simulink model "vertical_smm_3d_with_xz_lqr"  (R2015a)
settings: Solver=FixedStepDiscrete  SolverMode=SingleTasking  StartTime=0.0  StopTime=inf  FixedStep=sample_time  RelTol=1e-3
values from neighbouring files (symbols this model uses):
  forward_dx_of_dxstar = [-1.33773437568 -1.28773437515 -1.23773437461 -1.18773437408 -1.13773437355 -1.08773437301 -1.03773437248 -0.987734371946 -0.937734371413 -0.887734370879 -0.837734370532 -0.787734370254 ... (27552 elements, 41x21x32)]    [ref_trajs.mat]
  forward_x_of_dxstar = [0.243075305346 0.235858801492 0.228642297639 0.221425793786 0.214209289933 0.206992786079 0.199776282226 0.192559778373 0.18534327452 0.178126770666 0.17091026684 0.163693763058 ... (27552 elements, 41x21x32)]    [ref_trajs.mat]
  target_dx_range = [-1 -0.95 -0.9 -0.85 -0.8 -0.75 -0.7 -0.65 -0.6 -0.55 -0.5 -0.45 ... (41 elements, 1x41)]    [ref_trajs.mat]
undefined symbols (not defined in the file or in its folder): A1_notch_f1, A2_notch_f1, A_kalman_fourbar_gear, A_kalman_swing_load, A_kalman_transverse, A_kalman_vertical, A_lpf_accelerometer, A_lpf_dtau, A_lpf_fourbar_angles, A_lpf_imu, A_lpf_lateral_angle, B1_lpf_accelerometer, B1_lpf_dtau, B1_lpf_fourbar_angles, B1_lpf_imu, B1_lpf_lateral_angle, B1_notch_f1, B2_lpf_accelerometer, B2_lpf_dtau, B2_lpf_fourbar_angles, B2_lpf_imu, B2_lpf_lateral_angle, B2_notch_f1, B_dx_versus_x0, B_kalman_fourbar_gear, B_kalman_swing_load, B_kalman_transverse, B_kalman_vertical, backwards_K_sag_of_t, backwards_P_sag_of_t, C_kalman_fourbar_gear, C_kalman_swing_load, C_kalman_transverse, C_kalman_vertical, com_leg_motor, com_torso, contact_threshold, control_start_time, d_ankle_to_foot, d_vertical_com, desired_com_forward_velocity, desired_com_lateral_velocity, desired_initial_leg_roll_left, desired_initial_leg_roll_right, desired_stance_beta2, desired_standing_torso_pitch, desired_standing_torso_roll, desired_standing_z, desired_torso_pitch, desired_torso_roll, Discrete, enable_bouncing, fcut_contact, fdesignblkfcn, g, gcbh, HIP_MTR_MAX_CONT_TORQUE, HIP_MTR_MAX_TORQUE, i_leg_motor, i_robot ... (+91)
libraries: simulink x33, ctrlSharedLib x11, dsparch4 x10, dspfdesign x2
(part 5 of 7)

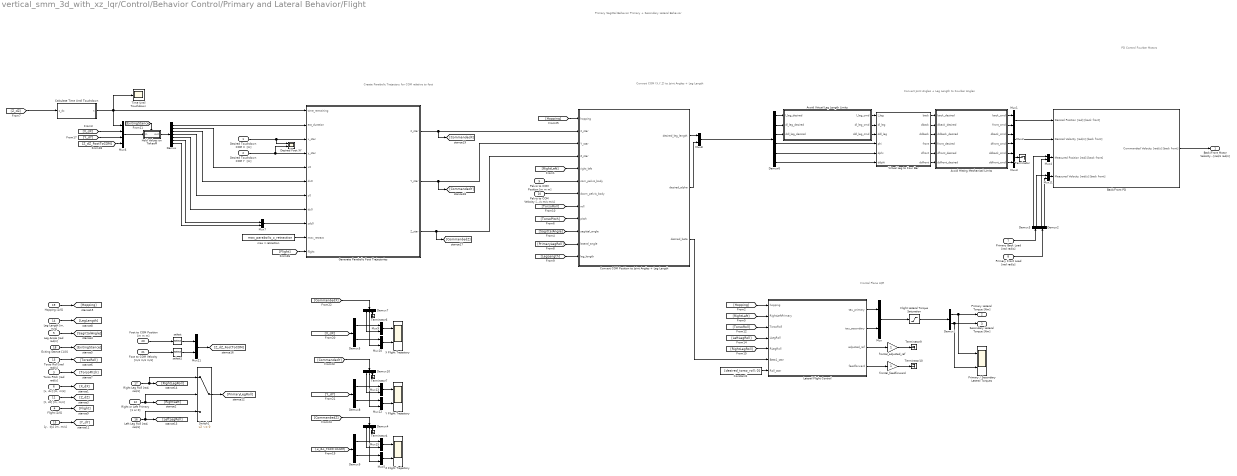
== system vertical_smm_3d_with_xz_lqr/Control/Behavior Control/Primary and Lateral Behavior/Flight ==
  note: Frontal Plane LQR
  note: PD Control Fourbar Motors
  note: Convert Joint Angles + Leg Length
      | to Fourbar Angles
  note: Convert COM (X,Y,Z) to
      | Joint Angles + Leg Length
  note: Create Parabolic
      | Trajectory for COM relative to foot
  note: Primary Sagittal Behavior
      | Primary + Secondary Lateral Behavior
  Desired Touchdown COM X  [m] : Inport
  Desired Touchdown COM Y  [m] : Inport  Port=2
  Torso Pitch [rad rad/s] : Inport  Port=3
  Flight [1/0] : Inport  Port=4
  Leg Angle [rad rad/s] : Inport  Port=5
  "[x, dx] [m, m/s]" : Inport  Port=6
  Primary Back Load [rad rad/s] : Inport  Port=7
  Primary Front Load [rad rad/s] : Inport  Port=8
  Pelvis to COM Position [m m m] : Inport  Port=9
  Pelvis to COM Velocity [m/s m/s m/s] : Inport  Port=10
  "[z, dz] [m, m/s]" : Inport  Port=11
  Right or Left Primary [1 or 0] : Inport  Port=12
  Torso Roll [rad rad/s] : Inport  Port=13
  "Leg Length [m, m/s]" : Inport  Port=14
  "[y,  dy] [m, m/s]" : Inport  Port=15
  "Left Leg Roll [rad, rad/s]" : Inport  Port=16
  "Right Leg Roll [rad, rad/s]" : Inport  Port=17
  Exiting Stance [1/0] : Inport  Port=18
  Hopping [1/0] : Inport  Port=19
  Foot to COM Position [m m m] : Inport  Port=20
  Foot to COM Velocity [m/s m/s m/s] : Inport  Port=21
  Avoid Hitting Mechanical Limits : MATLAB Function  TreatAsAtomicUnit=on
  Avoid Virtual Leg Length Limits : MATLAB Function  TreatAsAtomicUnit=on
  Back/Front PD : Subsystem
  Calculate Time Until Touchdown : MATLAB Function  TreatAsAtomicUnit=on
  Constant1 : Constant  Value=[desired_torso_roll; 0]
  "Convert COM Position to Joint Angles + Leg Length " : MATLAB Function  TreatAsAtomicUnit=on
  Demux : Demux  Outputs=7
  Demux{1..3,5,8..9} (6 alike) : Demux  Outputs=2
  Demux10 : Demux  Outputs=3
  Demux4 : Demux  Outputs=3
  Demux6 : Demux  Outputs=6
  Demux7 : Demux  Outputs=3
  Desired Foot XY : Scope  NumInputPorts=2
      settings: YMin=-1~-0.8  YMax=1~1.4  SaveName=ScopeData38  SampleInput=on
  Flight Lateral Torque Saturation : Saturate  UpperLimit=HIP_MTR_MAX_CONT_TORQUE  LowerLimit=-HIP_MTR_MAX_CONT_TORQUE
      settings: AttributesFormatString=Top: %<UpperLimit>\nBottom: %<LowerLimit>
  Generate Parabolic Foot Trajectories : MATLAB Function  TreatAsAtomicUnit=on
  Hold Values on Takeoff : Subsystem
  Lateral Flight Control : MATLAB Function  TreatAsAtomicUnit=on
  Mux{,1..5,7..13,15,21} (15 alike) : Mux  Inputs=2
  Mux6 : Mux
  Primary / Secondary Lateral Torques : Scope  NumInputPorts=2
      settings: YMin=-1~-0.8  YMax=1~1.4  SaveName=ScopeData32  SampleInput=on
  Switch1 : Switch  Criteria=u2 ~= 0
  Terminator{,4,6..7,9..10} (6 alike) : Terminator
  Time Until Touchdown : Scope
      settings: YMin=-1  YMax=1  SaveName=ScopeData37  SampleInput=on
  Virtual Leg to Four Bar : MATLAB Function  TreatAsAtomicUnit=on
  X Flight Trajectory : Scope  NumInputPorts=2
      settings: YMin=-1~-0.8  YMax=1~1.4  SaveName=ScopeData3  SampleInput=on
  Y Flight Trajectory : Scope  NumInputPorts=2
      settings: YMin=-1~-0.8  YMax=1~1.4  SaveName=ScopeData4  SampleInput=on
  Z Flight Trajectory : Scope  NumInputPorts=2
      settings: YMin=-1~-0.8  YMax=1~1.4  SaveName=ScopeData7  SampleInput=on
  frontal_adjusted_ref : Gain
  frontal_feedforward : Gain
  max z retraction : Constant  Value=max_parabolic_z_retraction
  select : Selector  InputPortWidth=3  Indices=[3]
  select1 : Selector  InputPortWidth=3  Indices=[3]
  Back/Front Motor Velocity [rad/s rad/s] : Outport
  Primary Lateral Torque [Nm] : Outport  Port=2
  Secondary Lateral Torque [Nm] : Outport  Port=3
  wires:
  Mux3/1 -> Terminator/1
  Generate Parabolic Foot Trajectories/3(Z_star) -> [CommandedZ], "Convert COM Position to Joint Angles + Leg Length "/4(Z_star)
  [CommandedZ] -> Demux4/1
  [CommandedY] -> Demux10/1
  [CommandedX] -> Demux7/1
  Demux10/3 -> Terminator7/1
  [Y_dY] -> Demux8/1
  Demux10/2 -> Mux12/2
  Demux10/1 -> Mux13/2
  Demux8/2 -> Mux12/1
  Demux8/1 -> Mux13/1
  Mux12/1 -> Y Flight Trajectory/2
  Mux13/1 -> Y Flight Trajectory/1
  Demux7/3 -> Terminator6/1
  [X_dX] -> Demux5/1
  Demux7/2 -> Mux10/2
  Demux7/1 -> Mux9/2
  Demux5/2 -> Mux10/1
  Demux5/1 -> Mux9/1
  Mux10/1 -> X Flight Trajectory/2
  Mux9/1 -> X Flight Trajectory/1
  Demux4/3 -> Terminator4/1
  Demux4/2 -> Mux5/2
  Demux4/1 -> Mux15/2
  Demux9/2 -> Mux5/1
  Demux9/1 -> Mux15/1
  [Z_dZ_FootToCOM] -> Demux9/1
  [Z_dZ_FootToCOM] -> Mux6/4
  Mux5/1 -> Z Flight Trajectory/2
  Mux15/1 -> Z Flight Trajectory/1
  Mux21/1 -> [Z_dZ_FootToCOM]
  select1/1 -> Mux21/2
  select/1 -> Mux21/1
  Foot to COM Velocity [m/s m/s m/s]/1 -> select1/1
  Foot to COM Position [m m m]/1 -> select/1
  Demux/7 -> Mux7/2
  Demux/6 -> Mux7/1
  Demux/5 -> Generate Parabolic Foot Trajectories/8(dy0)
  Demux/4 -> Generate Parabolic Foot Trajectories/7(y0)
  Demux/3 -> Generate Parabolic Foot Trajectories/6(dx0)
  Demux/2 -> Generate Parabolic Foot Trajectories/5(x0)
  [Flight] -> Generate Parabolic Foot Trajectories/11(flight)
  Hopping [1/0]/1 -> [Hopping]
  [Hopping] -> Lateral Flight Control/1(hopping)
  Mux/1 -> Flight Lateral Torque Saturation/1
  [Hopping] -> "Convert COM Position to Joint Angles + Leg Length "/1(hopping)
  frontal_adjusted_ref/1 -> Terminator9/1
  frontal_feedforward/1 -> Terminator10/1
  Flight Lateral Torque Saturation/1 -> Demux1/1
  "Convert COM Position to Joint Angles + Leg Length "/3(desired_beta) -> Lateral Flight Control/6(Beta1_star)
  Demux1/2 -> Secondary Lateral Torque [Nm]/1, Primary / Secondary Lateral Torques/2
  Demux1/1 -> Primary Lateral Torque [Nm]/1, Primary / Secondary Lateral Torques/1
  Exiting Stance [1/0]/1 -> [ExitingStance]
  Switch1/1 -> [PrimaryLegRoll]
  Right or Left Primary [1 or 0]/1 -> [RightLeft], Switch1/2
  "Right Leg Roll [rad, rad/s]"/1 -> [RightLegRoll], Switch1/1
  [RightLegRoll] -> Lateral Flight Control/5(RLegRoll)
  [LeftLegRoll] -> Lateral Flight Control/4(LLegRoll)
  "Left Leg Roll [rad, rad/s]"/1 -> [LeftLegRoll], Switch1/3
  Lateral Flight Control/1(tau_primary) -> Mux/1
  Lateral Flight Control/2(tau_secondary) -> Mux/2
  Lateral Flight Control/4(feedforward) -> frontal_feedforward/1
  Lateral Flight Control/3(adjusted_ref) -> frontal_adjusted_ref/1
  Constant1/1 -> Lateral Flight Control/7(Roll_star)
  [TorsoRoll] -> Lateral Flight Control/3(TorsoRoll)
  [RightLeft] -> Lateral Flight Control/2(RightLeftPrimary)
  Desired Touchdown COM Y  [m]/1 -> Generate Parabolic Foot Trajectories/4(y_star), Desired Foot XY/2
  Demux6/3 -> Avoid Virtual Leg Length Limits/3(ddl_leg_desired)
  Demux6/2 -> Avoid Virtual Leg Length Limits/2(dl_leg_desired)
  Demux6/1 -> Avoid Virtual Leg Length Limits/1(l_leg_desired)
  Avoid Virtual Leg Length Limits/3(ddl_leg_cmd) -> Virtual Leg to Four Bar/3(ddl_leg)
  Avoid Virtual Leg Length Limits/2(dl_leg_cmd) -> Virtual Leg to Four Bar/2(dl_leg)
  Avoid Virtual Leg Length Limits/1(l_leg_cmd) -> Virtual Leg to Four Bar/1(l_leg)
  Calculate Time Until Touchdown/1(t) -> Generate Parabolic Foot Trajectories/1(time_remaining), Time Until Touchdown/1, Mux6/1
  [Z_dZ] -> Calculate Time Until Touchdown/1(z_dz)
  [Y_dY] -> Mux6/3
  "[y,  dy] [m, m/s]"/1 -> [Y_dY]
  Desired Touchdown COM X  [m]/1 -> Generate Parabolic Foot Trajectories/3(x_star), Desired Foot XY/1
  "[z, dz] [m, m/s]"/1 -> [Z_dZ]
  "Leg Length [m, m/s]"/1 -> [LegLength]
  Torso Roll [rad rad/s]/1 -> [TorsoRoll]
  "[x, dx] [m, m/s]"/1 -> [X_dX]
  [ExitingStance] -> Hold Values on Takeoff/Trigger
  Flight [1/0]/1 -> [Flight]
  Pelvis to COM Velocity [m/s m/s m/s]/1 -> "Convert COM Position to Joint Angles + Leg Length "/7(dcom_pelvis_body)
  Pelvis to COM Position [m m m]/1 -> "Convert COM Position to Joint Angles + Leg Length "/6(com_pelvis_body)
  [TorsoRoll] -> "Convert COM Position to Joint Angles + Leg Length "/8(roll)
  [LegLength] -> "Convert COM Position to Joint Angles + Leg Length "/12(leg_length)
  [PrimaryLegRoll] -> "Convert COM Position to Joint Angles + Leg Length "/11(lateral_angle)
  [TorsoPitch] -> "Convert COM Position to Joint Angles + Leg Length "/9(pitch)
  Torso Pitch [rad rad/s]/1 -> [TorsoPitch]
  [SagittalAngle] -> "Convert COM Position to Joint Angles + Leg Length "/10(sagittal_angle)
  Leg Angle [rad rad/s]/1 -> [SagittalAngle]
  Mux8/1 -> Demux6/1
  Demux6/4 -> Virtual Leg to Four Bar/4(phi)
  Demux6/5 -> Virtual Leg to Four Bar/5(dphi)
  Demux6/6 -> Virtual Leg to Four Bar/6(ddphi)
  "Convert COM Position to Joint Angles + Leg Length "/1(desired_leg_length) -> Mux8/1
  "Convert COM Position to Joint Angles + Leg Length "/2(desired_alpha) -> Mux8/2
  [RightLeft] -> "Convert COM Position to Joint Angles + Leg Length "/5(right_left)
  Generate Parabolic Foot Trajectories/2(Y_star) -> [CommandedY], "Convert COM Position to Joint Angles + Leg Length "/3(Y_star)
  Generate Parabolic Foot Trajectories/1(X_star) -> "Convert COM Position to Joint Angles + Leg Length "/2(X_star), [CommandedX]
  [X_dX] -> Mux6/2
  Hold Values on Takeoff/1(out) -> Demux/1
  Mux6/1 -> Hold Values on Takeoff/1(in)
  max z retraction/1 -> Generate Parabolic Foot Trajectories/10(max_retract)
  Mux7/1 -> Generate Parabolic Foot Trajectories/9(zdz0)
  Demux/1 -> Generate Parabolic Foot Trajectories/2(est_duration)
  Primary Front Load [rad rad/s]/1 -> Demux2/1
  Primary Back Load [rad rad/s]/1 -> Demux3/1
  Back/Front PD/1(Commanded Velocity [rad/s] [back front]) -> Back/Front Motor Velocity [rad/s rad/s]/1
  Mux2/1 -> Back/Front PD/2(Desired Velocity [rad/s] [back front])
  Avoid Hitting Mechanical Limits/6(ddfront_cmd) -> Mux3/2
  Avoid Hitting Mechanical Limits/5(ddback_cmd) -> Mux3/1
  Avoid Hitting Mechanical Limits/4(dfront_cmd) -> Mux2/2
  Avoid Hitting Mechanical Limits/3(dback_cmd) -> Mux2/1
  Demux2/1 -> Mux4/2
  Avoid Hitting Mechanical Limits/1(back_cmd) -> Mux1/1
  Avoid Hitting Mechanical Limits/2(front_cmd) -> Mux1/2
  Demux3/1 -> Mux4/1
  Demux3/2 -> Mux11/1
  Mux1/1 -> Back/Front PD/1(Desired Position [rad] [back front])
  Mux4/1 -> Back/Front PD/3(Measured Position [rad] [back front])
  Demux2/2 -> Mux11/2
  Mux11/1 -> Back/Front PD/4(Measured Velocity [rad/s] [back front])
  Virtual Leg to Four Bar/6(ddfront) -> Avoid Hitting Mechanical Limits/6(ddfront_desired)
  Virtual Leg to Four Bar/5(dfront) -> Avoid Hitting Mechanical Limits/5(dfront_desired)
  Virtual Leg to Four Bar/4(front) -> Avoid Hitting Mechanical Limits/4(front_desired)
  Virtual Leg to Four Bar/3(ddback) -> Avoid Hitting Mechanical Limits/3(ddback_desired)
  Virtual Leg to Four Bar/2(dback) -> Avoid Hitting Mechanical Limits/2(dback_desired)
  Virtual Leg to Four Bar/1(back) -> Avoid Hitting Mechanical Limits/1(back_desired)

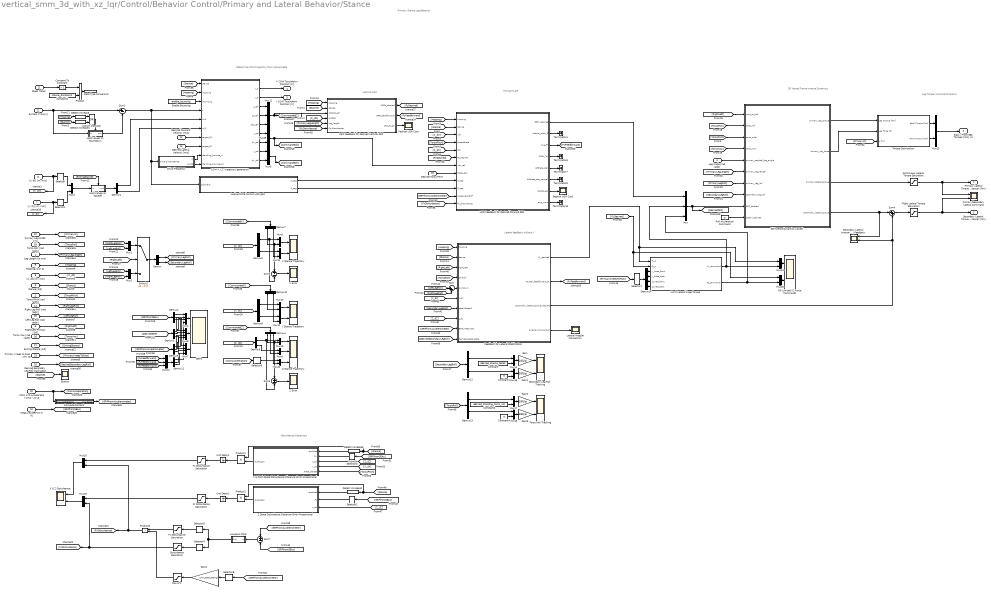
== system vertical_smm_3d_with_xz_lqr/Control/Behavior Control/Primary and Lateral Behavior/Stance ==
  note: Leg Torque / Force
      | Distribution
  note: Disturbance Observers
  note: Primary Stance Leg Behavior
  note: Determine COM trajectory
      | from lookup table
  note: Vertical LQR
  note: Forward LQR
  note: 3D Yawed Frame Inverse Dynamics
  note: Lateral feedback without Y
  Leg Length [m m/s] : Inport
  Torso Pitch [rad rad/s] : Inport  Port=2
  Stance [1/0] : Inport  Port=3
  Leg Angle [rad rad/s] : Inport  Port=4
  Right/Left Primary [1/0] : Inport  Port=5
  "[x, dx] [m, m/s]" : Inport  Port=6
  "[y, dy] [m, m/s]" : Inport  Port=7
  "[z, dz] [m, m/s]" : Inport  Port=8
  Hopping [1 or 0] : Inport  Port=9
  Measured GRF [N N N] : Inport  Port=10
  Steps Taken : Inport  Port=11
  Desired Forward Velocity [m/s] : Inport  Port=12
  Desired Lateral Velocity [m/s] : Inport  Port=13
  Right Leg Roll [rad rad/s] : Inport  Port=14
  Left Leg Roll [rad rad/s] : Inport  Port=15
  Torso Yaw [rad rad/s] : Inport  Port=16
  Exiting Stance [1/0] : Inport  Port=17
  Desired Torso Pitch : Inport  Port=18
  Torso Roll [rad rad/s] : Inport  Port=19
  COM XYZ Acceleration [m/s^2] x3 : Inport  Port=20
  System Time [s] : Inport  Port=21
  Primary Leg Width [m] : Inport  Port=22
  Primary Knees to Foot [m] x6 : Inport  Port=23
  Desired Secondary Leg Roll [rad rad/s] : Inport  Port=24
  3D Inverse Dynamics yawed : MATLAB Function  TreatAsAtomicUnit=on
  COM X,Y,Z  trajectory generation : MATLAB Function  TreatAsAtomicUnit=on
  Chirp Frequency : Subsystem
  Compare To Constant : simulink/Logic and Bit Operations/Compare To Constant  relop=<  const=1  OutDataTypeStr=uint8
  Compute Forces1 : Subsystem
  Constant : Constant  Value=desired_stance_beta2
  Constant1 : Constant  Value=0
  Constant2 : Constant  Value=stance_duration/2
  Constant3 : Constant  Value=desired_standing_torso_roll
  Constant4 : Constant  Value=0
  Continuous Lateral Torque Saturation : Saturate  UpperLimit=max_primary_lateral_stance_torque  LowerLimit=-max_primary_lateral_stance_torque
      settings: AttributesFormatString=Top: %<UpperLimit>\nBottom: %<LowerLimit>
  Data Type Conversion : DataTypeConversion  OutDataTypeStr=double
  Demux{,1,5,7..10,12..13} (9 alike) : Demux  Outputs=2
  Demux{2..4,6,11} (5 alike) : Demux  Outputs=3
  Demux14 : Demux
  Detect Increase{,1..3} (4 alike) : simulink/Logic and Bit Operations/Detect Increase  vinit=0.0  InputProcessing=Inherited  OutDataTypeStr=boolean
  "Disturbance Saturation " : Saturate  UpperLimit=100  LowerLimit=-100
      settings: AttributesFormatString=Top: %<UpperLimit>\nBottom: %<LowerLimit>
  Enable Bouncing : Constant  Value=enable_bouncing  SampleTime=sample_time
  Feedback for Lateral Stabilization : MATLAB Function  TreatAsAtomicUnit=on
  Flight Lateral Torque Saturation : Saturate  UpperLimit=HIP_MTR_MAX_CONT_TORQUE  LowerLimit=-HIP_MTR_MAX_CONT_TORQUE
      settings: AttributesFormatString=Top: %<UpperLimit>\nBottom: %<LowerLimit>
  Fx Disturbance Saturation : Saturate  UpperLimit=100  LowerLimit=-100
      settings: AttributesFormatString=Top: %<UpperLimit>\nBottom: %<LowerLimit>
  "Fx Disturbance Saturation " : Saturate  UpperLimit=100  LowerLimit=-100
      settings: AttributesFormatString=Top: %<UpperLimit>\nBottom: %<LowerLimit>
  Fz Disturbance Saturation : Saturate  UpperLimit=100  LowerLimit=-100
      settings: AttributesFormatString=Top: %<UpperLimit>\nBottom: %<LowerLimit>
  GRFs : Scope  NumInputPorts=3
      settings: TimeRange=37.999  YMin=-1250~-2000~-1250  YMax=1500~3750~1750  SampleInput=on
  Gain{,1..3} (4 alike) : Gain  Gain=180/pi
  Gain4 : Gain  Gain=2/(m_total_real*g)
  Hold Values on Takeoff : Subsystem
  Hold Values on Touchdown : Subsystem
  LQR Feedback for Desired Forward GRF : MATLAB Function  TreatAsAtomicUnit=on
  LQR Feedback for Desired Vertical GRF : MATLAB Function  TreatAsAtomicUnit=on
  Lateral Angular Momentum : Scope
      settings: YMin=-3.5  YMax=4  SaveName=ScopeData20  SampleInput=on
  Limit Lateral Knee Torque : MATLAB Function  TreatAsAtomicUnit=on
  Logical Operator : Logic  Operator=OR  AllPortsSameDT=off  OutDataTypeStr=boolean
  Lookup finite horizon LQR gain : MATLAB Function  TreatAsAtomicUnit=on
  Lowpass Filter : Subsystem  DialogController=fdesignblkfcn  InitFcn=fdesignblkfcn(gcbh, {'InitFcn'});  mask(Lowpass Filter){}
      mask help: Design a lowpass filter
      settings: CopyFcn=fdesignblkfcn(gcbh, {'CopyFcn'});
      mask Help: helpview(mapfilelocation('dsp'), 'dsplowpassfilter');
      mask Display: disp('Lowpass')
  Max of 1 : Saturate  UpperLimit=1  LowerLimit=0
      settings: AttributesFormatString=Top: %<UpperLimit>\nBottom: %<LowerLimit>
  Mux : Mux  Inputs=3
  Mux{1..3,5,8..10,12..20,22..25,49} (21 alike) : Mux  Inputs=2
  Mux11 : Mux  Inputs=3
  Mux21 : Mux  Inputs=3
  Mux4 : Mux
  Mux6 : Mux
  Mux7 : Mux
  Primary/Secondary Lateral Command : Scope  NumInputPorts=2
      settings: YMin=40~-5  YMax=150~5  SaveName=ScopeData25  SampleInput=on
  Product{,1..3} (4 alike) : Product
  QP Limited YZ Force Commands : Scope  NumInputPorts=2
      settings: YMin=40~-5  YMax=150~5  SaveName=ScopeData26  SampleInput=on
  Roll Accleration Command : Constant  Value=0
  Sagittal LQR Cost : Scope
      settings: YMin=22.5  YMax=62.5  SaveName=ScopeData10  SampleInput=on
  Secondary Lateral Inverse Dynamics / Feedback : Scope  NumInputPorts=2
      settings: YMin=-3.5~-5  YMax=4~5  SaveName=ScopeData9  SampleInput=on
  Secondary Leg Roll Tracking : Scope  NumInputPorts=2
      settings: YMin=-3.5~-5  YMax=4~5  SaveName=ScopeData12  SampleInput=on
  Selector : Selector  InputPortWidth=2  Indices=[2]
  Selector1 : Selector  InputPortWidth=2  Indices=[2]
  Selector{2,4,6,8} (4 alike) : Selector  InputPortWidth=3  Indices=[3]
  Selector3 : Selector  InputPortWidth=3  Indices=[1]
  Selector5 : Selector  InputPortWidth=3  Indices=[1]
  Selector7 : Selector  InputPortWidth=6  Indices=[2 5 3 6]
  Stance : Scope
      settings: YMin=-0.05  YMax=0.11  SaveName=stance_time_history  SampleInput=on
  Sum : Sum  Inputs=|+-
  Sum2 : Sum  Inputs=|+-
  Sum4 : Sum  Inputs=|++
  Sum5 : Sum  Inputs=+-
  Sum6 : Sum  Inputs=+-
  Sum7 : Sum  Inputs=+-
  Switch1 : Switch  Criteria=u2 ~= 0
  Terminator{4,6..8,10} (5 alike) : Terminator
  Torque Distribution : Subsystem
  Torso Roll Tracking : Scope  NumInputPorts=2
      settings: YMin=-3.5~-5  YMax=4~5  SaveName=ScopeData15  SampleInput=on
  Unit Delay1 : UnitDelay  SampleTime=sample_time
  Unit Delay2 : UnitDelay  SampleTime=sample_time
  Vertical LQR Cost : Scope
      settings: YMin=11  YMax=16  SaveName=ScopeData18  SampleInput=on
  X & Pitch State Disturbance Observer Error-Proportional : MATLAB Function  TreatAsAtomicUnit=on
  X & Z Disturbance : Scope  NumInputPorts=2
      settings: YMin=-125~-800  YMax=175~700  SaveName=ScopeData16  SampleInput=on
  X Stance Trajectory : Scope  NumInputPorts=2
      settings: YMin=0~-0.02  YMax=0.005~0.03  SaveName=ScopeData8  SampleInput=on
  X error : Scope
      settings: YMin=-0.05  YMax=0.11  SaveName=ScopeData24  SampleInput=on
  Y Stance Trajectory : Scope  NumInputPorts=2
      settings: YMin=0.005~-0.5  YMax=0.1~0.3  SaveName=ScopeData5  SampleInput=on
  Z Error : Scope
      settings: YMin=-0.007  YMax=0.0005  SaveName=ScopeData23  SampleInput=on
  Z Stance Trajectory : Scope  NumInputPorts=3
      settings: YMin=0.85~-0.4~-3  YMax=0.98~0.6~11  SaveName=z_stance_trajectory  SampleInput=on
  Z State Disturbance Observer Error-Proportional : MATLAB Function  TreatAsAtomicUnit=on
  Primary Lateral Torque Command (stance) [Nm] : Outport
  Secondary Lateral Torque Command (stance) [Nm] : Outport  Port=2
  Back / Front SEA Torques [Nm] x2 : Outport  Port=3
  X COM Touchdown Position [m] : Outport  Port=4
  Y COM Touchdown Position [m] : Outport  Port=5
  wires:
  Limit Lateral Knee Torque/1(Fy_command) -> Mux/2, Mux24/2
  Mux25/1 -> QP Limited YZ Force Commands/2
  Mux24/1 -> QP Limited YZ Force Commands/1
  Selector7/1 -> Demux14/1
  Demux14/4 -> Limit Lateral Knee Torque/6(z_knee_back)
  Demux14/3 -> Limit Lateral Knee Torque/5(z_knee_front)
  Demux14/2 -> Limit Lateral Knee Torque/4(y_knee_back)
  Demux14/1 -> Limit Lateral Knee Torque/3(y_knee_front)
  [PrimaryKneesToFoot] -> Selector7/1
  Primary Knees to Foot [m] x6/1 -> [PrimaryKneesToFoot]
  Feedback for Lateral Stabilization/2(neutral_feedforward_Fy) -> [FyFeedforward]
  LQR Feedback for Desired Forward GRF/2(netural_pitch_ff) -> Terminator4/1
  LQR Feedback for Desired Forward GRF/3(true_ff) -> [FxFeedforward]
  Compute Forces1/1(XYZ Force) -> [GRFfromAccelerometer]
  [FyFeedforward] -> Mux21/2
  [Z_dZ] -> Feedback for Lateral Stabilization/8(z_dz)
  [FzDesired] -> Mux25/1, Limit Lateral Knee Torque/2(Fz_s)
  [FzDesired] -> LQR Feedback for Desired Forward GRF/6(Fz_desired)
  [FxFeedforward] -> Mux21/1
  Mux23/1 -> Back / Front SEA Torques [Nm] x2/1
  Torque Distribution/2(Front Torque [Nm]) -> Mux23/2
  Torque Distribution/1(Back Torque [Nm]) -> Mux23/1
  Primary Leg Width [m]/1 -> [PrimaryW]
  3D Inverse Dynamics yawed/2(primary_leg_force) -> Torque Distribution/2(Leg Force [N])
  [PrimaryW] -> Torque Distribution/3(w [m])
  3D Inverse Dynamics yawed/1(primary_leg_torque) -> Torque Distribution/1(Leg Torque [Nm])
  Selector6/1 -> Mux22/1
  [ComAcceleration] -> Selector6/1
  Mux22/1 -> Z Stance Trajectory/3
  Sum5/1 -> Z Error/1
  [CommandedZ] -> Demux4/1
  Demux4/3 -> Mux22/2
  Demux4/2 -> Mux8/2
  Demux4/1 -> Sum5/1, Mux15/2
  Demux9/2 -> Mux8/1
  Demux9/1 -> Sum5/2, Mux15/1
  [Z_dZ] -> Demux9/1
  Mux8/1 -> Z Stance Trajectory/2
  Mux15/1 -> Z Stance Trajectory/1
  [FzFeedforward] -> Mux21/3
  Mux21/1 -> Demux11/1
  LQR Feedback for Desired Vertical GRF/2(GRFz_feedforward) -> [FzFeedforward]
  [GRFfromAccelerometer] -> Demux6/1
  COM XYZ Acceleration [m/s^2] x3/1 -> [ComAcceleration], Compute Forces1/1(XYZ Acceleration)
  Selector4/1 -> "Disturbance Saturation "/1
  [GRFfromSEAs] -> Sum7/2
  Mux19/1 -> X & Z Disturbance/2
  [Stance] -> Detect Increase2/1, Product2/1
  Z State Disturbance Observer Error-Proportional/1(d_hat_tp1) -> Product2/2
  [Stance] -> Detect Increase3/1, Product1/1
  X & Pitch State Disturbance Observer Error-Proportional/1(d_hat_tp1) -> Product1/2
  Product2/1 -> Unit Delay2/1
  Product1/1 -> Unit Delay1/1
  [Z_dZ] -> Z State Disturbance Observer Error-Proportional/3(z_dz)
  [GRFfromSEAs] -> Selector2/1
  Detect Increase2/1 -> Z State Disturbance Observer Error-Proportional/1(enabled)
  Detect Increase3/1 -> X & Pitch State Disturbance Observer Error-Proportional/1(enabled)
  [GRFfromSEAs] -> Selector3/1
  [X_dX] -> X & Pitch State Disturbance Observer Error-Proportional/4(x_dx)
  [TorsoPitch] -> X & Pitch State Disturbance Observer Error-Proportional/5(theta_dtheta)
  [Z_dZ] -> X & Pitch State Disturbance Observer Error-Proportional/3(z_dz)
  "[z, dz] [m, m/s]"/1 -> [Z_dZ]
  Flight Lateral Torque Saturation/1 -> Secondary Lateral Torque Command (stance) [Nm]/1, Primary/Secondary Lateral Command/2
  Demux6/3 -> Mux7/3
  Demux6/2 -> Mux6/3
  Demux6/1 -> Mux4/3
  Feedback for Lateral Stabilization/4(angular_momentum) -> Lateral Angular Momentum/1
  LQR Feedback for Desired Forward GRF/4(GRFx_lqr) -> Terminator6/1
  [Stance] -> COM X,Y,Z  trajectory generation/1(stance)
  Lookup finite horizon LQR gain/2(P_sag) -> LQR Feedback for Desired Forward GRF/10(P_sag)
  [Z_dZ] -> LQR Feedback for Desired Vertical GRF/4(z_state)
  COM X,Y,Z  trajectory generation/3(z_ref) -> Mux11/1
  [Stance] -> LQR Feedback for Desired Forward GRF/2(stance)
  COM X,Y,Z  trajectory generation/6(x_ref) -> Mux49/1
  COM X,Y,Z  trajectory generation/7(dx_ref) -> Mux49/2
  COM X,Y,Z  trajectory generation/8(y_ref) -> Mux5/1
  COM X,Y,Z  trajectory generation/9(dy_ref) -> Mux5/2
  COM X,Y,Z  trajectory generation/1(x_0) -> X COM Touchdown Position [m]/1
  COM X,Y,Z  trajectory generation/4(dz_ref) -> Mux11/2
  COM X,Y,Z  trajectory generation/5(ddz_ref) -> Mux11/3
  Mux11/1 -> [CommandedZ], LQR Feedback for Desired Vertical GRF/3(zdzddz_ref)
  [X_dX] -> LQR Feedback for Desired Forward GRF/3(xdx)
  [TorsoPitch] -> LQR Feedback for Desired Forward GRF/4(thetadtheta)
  Mux49/1 -> [CommandedX], LQR Feedback for Desired Forward GRF/7(xdx_ref)
  Desired Torso Pitch/1 -> LQR Feedback for Desired Forward GRF/8(theta_star)
  Lookup finite horizon LQR gain/1(K_sag) -> LQR Feedback for Desired Forward GRF/9(K_sag)
  [Z_dZ] -> LQR Feedback for Desired Forward GRF/5(zdz)
  Desired Forward Velocity [m/s]/1 -> COM X,Y,Z  trajectory generation/7(target_DX)
  Sum2/1 -> COM X,Y,Z  trajectory generation/4(t), Lookup finite horizon LQR gain/1(t_forward), Chirp Frequency/1(Time Since Stance)
  LQR Feedback for Desired Vertical GRF/1(GRFz_desired) -> [FzDesired]
  Hold Values on Touchdown/1(out) -> Sum2/2
  Stance [1/0]/1 -> [Stance]
  [Stance] -> LQR Feedback for Desired Vertical GRF/2(stance)
  Logical Operator/1 -> Hold Values on Touchdown/Trigger
  "[x, dx] [m, m/s]"/1 -> [X_dX], Selector/1
  Demux1/2 -> COM X,Y,Z  trajectory generation/6(dy0)
  LQR Feedback for Desired Vertical GRF/3(cost_to_go) -> Vertical LQR Cost/1
  LQR Feedback for Desired Forward GRF/5(ddtheta_star) -> Terminator7/1
  LQR Feedback for Desired Forward GRF/6(ddtheta_star_neutral) -> Terminator8/1
  LQR Feedback for Desired Forward GRF/7(cost_to_go) -> Sagittal LQR Cost/1
  LQR Feedback for Desired Forward GRF/8(ang_mom) -> Terminator10/1
  Torso Pitch [rad rad/s]/1 -> [TorsoPitch]
  [RightLeft] -> 3D Inverse Dynamics yawed/1(right_or_left)
  Hopping [1 or 0]/1 -> [Hopping]
  [Hopping] -> COM X,Y,Z  trajectory generation/2(hopping)
  [Hopping] -> LQR Feedback for Desired Forward GRF/1(hopping)
  Measured GRF [N N N]/1 -> [GRFfromSEAs]
  [GRFfromAccelerometer] -> LQR Feedback for Desired Forward GRF/11(measured_GRF)
  Steps Taken/1 -> Compare To Constant/1
  Product/1 -> Data Type Conversion/1
  Constant2/1 -> Product/2
  Detect Increase/1 -> Logical Operator/1
  Detect Increase1/1 -> Logical Operator/2
  Compare To Constant/1 -> Product/1
  [Hopping] -> Detect Increase/1
  [Stance] -> Detect Increase1/1
  Demux1/1 -> COM X,Y,Z  trajectory generation/5(dx0)
  Selector/1 -> Mux3/1
  [Hopping] -> LQR Feedback for Desired Vertical GRF/1(hopping)
  [Stance] -> Feedback for Lateral Stabilization/2(stance)
  [TorsoRoll] -> Feedback for Lateral Stabilization/4(rolldroll)
  COM X,Y,Z  trajectory generation/2(y_0) -> Y COM Touchdown Position [m]/1
  Mux5/1 -> [CommandedY]
  [TorsoPitch] -> 3D Inverse Dynamics yawed/3(torso_pitch)
  [TorsoRoll] -> 3D Inverse Dynamics yawed/2(torso_roll)
  [TorsoYaw] -> 3D Inverse Dynamics yawed/4(torso_yaw)
  [PrimaryLegLength] -> 3D Inverse Dynamics yawed/6(primary_leg_length)
  Leg Angle [rad rad/s]/1 -> 3D Inverse Dynamics yawed/5(primary_sagittal_leg_angle)
  [SecondaryLegRoll] -> 3D Inverse Dynamics yawed/8(secondary_leg_roll)
  [PrimaryLegRoll] -> 3D Inverse Dynamics yawed/7(primary_leg_roll)
  Switch1/1 -> Demux/1
  Demux/2 -> [SecondaryLegRoll]
  Demux/1 -> [PrimaryLegRoll]
  Mux1/1 -> Switch1/1
  Mux2/1 -> Switch1/3
  Right Leg Roll [rad rad/s]/1 -> [RightLegRoll]
  [RightLegRoll] -> Mux1/1
  [LeftLegRoll] -> Mux1/2
  [LeftLegRoll] -> Mux2/1
  [RightLegRoll] -> Mux2/2
  [RightLeft] -> Switch1/2
  "[y, dy] [m, m/s]"/1 -> [Y_dY], Selector1/1
  Mux3/1 -> Hold Values on Takeoff/1(in)
  Hold Values on Takeoff/1(out) -> Demux1/1
  Selector1/1 -> Mux3/2
  Desired Lateral Velocity [m/s]/1 -> COM X,Y,Z  trajectory generation/8(target_DY)
  Torso Yaw [rad rad/s]/1 -> [TorsoYaw]
  Exiting Stance [1/0]/1 -> [ExitingStance]
  [ExitingStance] -> Hold Values on Takeoff/Trigger
  [Hopping] -> Feedback for Lateral Stabilization/1(hopping)
  [GRFfromAccelerometer] -> Feedback for Lateral Stabilization/9(GRF_measured)
  System Time [s]/1 -> Hold Values on Touchdown/1(in), Sum2/1
  Leg Length [m m/s]/1 -> [PrimaryLegLength]
  [PrimaryLegLength] -> LQR Feedback for Desired Vertical GRF/5(leg_length)
  Torso Roll [rad rad/s]/1 -> [TorsoRoll]
  [GRFfromSEAs] -> Demux2/1
  [DesiredGRF] -> Demux3/1
  Mux4/1 -> GRFs/1
  Demux2/1 -> Mux4/1
  Mux6/1 -> GRFs/2
  Mux7/1 -> GRFs/3
  Demux2/2 -> Mux6/1
  Demux2/3 -> Mux7/1
  Demux3/1 -> Mux4/2
  Demux3/2 -> Mux6/2
  Demux3/3 -> Mux7/2
  Mux9/1 -> X Stance Trajectory/1
  Mux10/1 -> X Stance Trajectory/2
  Demux5/2 -> Mux10/1
  Demux7/2 -> Mux10/2
  [X_dX] -> Demux5/1
  Mux13/1 -> Y Stance Trajectory/1
  Mux12/1 -> Y Stance Trajectory/2
  Demux8/1 -> Mux13/1
  Demux8/2 -> Mux12/1
  Demux10/1 -> Mux13/2
  Demux10/2 -> Mux12/2
  [Y_dY] -> Demux8/1
  [CommandedX] -> Demux7/1
  [CommandedY] -> Demux10/1
  Right/Left Primary [1/0]/1 -> [RightLeft]
  Left Leg Roll [rad rad/s]/1 -> [LeftLegRoll]
  LQR Feedback for Desired Forward GRF/1(GRFx_desired) -> Mux/1
  Mux/1 -> 3D Inverse Dynamics yawed/9(GRF_desired), [DesiredGRF]
  Demux11/1 -> Mux4/4
  Demux11/2 -> Mux6/4
  Demux11/3 -> Mux7/4
  Continuous Lateral Torque Saturation/1 -> Primary Lateral Torque Command (stance) [Nm]/1, Primary/Secondary Lateral Command/1
  Feedback for Lateral Stabilization/1(Fy_desired) -> Mux24/1, Limit Lateral Knee Torque/1(Fy_s)
  Roll Accleration Command/1 -> 3D Inverse Dynamics yawed/10(ddRoll_desired)
  [LeftLegRoll] -> Sum/1
  [RightLegRoll] -> Sum/2
  [Y_dY] -> Feedback for Lateral Stabilization/6(y_dy)
  [SecondaryLegRoll] -> Feedback for Lateral Stabilization/7(beta2dbeta2)
  Sum/1 -> Feedback for Lateral Stabilization/5(symdsym)
  3D Inverse Dynamics yawed/4(secondary_lateral_torque) -> Sum4/1, Secondary Lateral Inverse Dynamics / Feedback/1
  3D Inverse Dynamics yawed/3(primary_lateral_torque) -> Continuous Lateral Torque Saturation/1
  Sum4/1 -> Flight Lateral Torque Saturation/1
  Feedback for Lateral Stabilization/3(secondary_lateral_torque_desired) -> Secondary Lateral Inverse Dynamics / Feedback/2, Sum4/2
  [SecondaryLegRoll] -> Demux12/1
  Mux14/1 -> Gain/1
  Demux12/1 -> Mux14/1
  Constant/1 -> Mux14/2
  Gain/1 -> Secondary Leg Roll Tracking/1
  Gain1/1 -> Secondary Leg Roll Tracking/2
  Mux16/1 -> Gain1/1
  Demux12/2 -> Mux16/1
  Constant1/1 -> Mux16/2
  [TorsoRoll] -> Demux13/1
  Gain2/1 -> Torso Roll Tracking/1
  Gain3/1 -> Torso Roll Tracking/2
  Mux17/1 -> Gain2/1
  Demux13/1 -> Mux17/1
  Constant3/1 -> Mux17/2
  Demux13/2 -> Mux18/1
  Mux18/1 -> Gain3/1
  Constant4/1 -> Mux18/2
  [RightLeft] -> Feedback for Lateral Stabilization/3(right_left)
  Enable Bouncing/1 -> COM X,Y,Z  trajectory generation/3(bouncing)
  Fx Disturbance Saturation/1 -> Mux20/1
  Selector3/1 -> X & Pitch State Disturbance Observer Error-Proportional/2(Fx)
  Unit Delay1/1 -> Fx Disturbance Saturation/1
  Unit Delay2/1 -> Fz Disturbance Saturation/1
  Demux5/1 -> Sum6/2, Mux9/1
  Demux7/1 -> Sum6/1, Mux9/2
  Sum6/1 -> X error/1
  [GRFfromAccelerometer] -> Sum7/1
  Mux20/1 -> X & Z Disturbance/1
  Product3/1 -> [FxDisturbance], Mux20/2
  Sum7/1 -> Lowpass Filter/1(In)
  Selector2/1 -> Z State Disturbance Observer Error-Proportional/2(Fz)
  Chirp Frequency/1(w) -> COM X,Y,Z  trajectory generation/9(standing_bounce_w)
  [Stance] -> Stance/1
  Chirp Frequency/2(dw/dt) -> COM X,Y,Z  trajectory generation/10(standing_bounce_dw)
  Lowpass Filter/1(Out) -> Selector4/1, Selector5/1
  [FxDisturbance] -> LQR Feedback for Desired Forward GRF/12(Fx_disturbance)
  [FzDisturbance] -> LQR Feedback for Desired Vertical GRF/6(Fz_disturbance)
  Limit Lateral Knee Torque/2(Fz_command) -> Mux25/2, Mux/3
  [GRFfromAccelerometer] -> Selector8/1
  Selector8/1 -> Gain4/1
  Gain4/1 -> Max of 1/1
  "Fx Disturbance Saturation "/1 -> Product3/1
  Max of 1/1 -> Product3/2
  "Disturbance Saturation "/1 -> Mux19/2, [FzDisturbance]
  Selector5/1 -> "Fx Disturbance Saturation "/1
  Fz Disturbance Saturation/1 -> Mux19/1
  [DesiredSecondaryLegRoll] -> Feedback for Lateral Stabilization/10(desired_beta2_state)
  Desired Secondary Leg Roll [rad rad/s]/1 -> [DesiredSecondaryLegRoll]

== system vertical_smm_3d_with_xz_lqr/Control/Behavior Control/Secondary Leg Behavior/Back//Front PD ==
  Desired Position [rad] [back front] : Inport
  Desired Velocity [rad/s] [back front] : Inport  Port=2
  Measured Position [rad] [back front] : Inport  Port=3
  Measured Velocity [rad/s] [back front] : Inport  Port=4
  Back Tracking : Scope  NumInputPorts=2
      settings: YMin=3.725~-1  YMax=4.05~0.9  SaveName=ScopeData6  SampleInput=on
  Front Tracking : Scope  NumInputPorts=2
      settings: YMin=-1~-0.8  YMax=1~1.4  SaveName=ScopeData31  SampleInput=on
  Kp_SEA_Trajectory : Constant  Value=kp_velocity_swing_trajectory
  Mux{1..2,12..13} (4 alike) : Mux  Inputs=2
  Product1 : Product
  Selector{,1..3} (4 alike) : Selector  InputPortWidth=2  Indices=[1]
  Selector{4..7} (4 alike) : Selector  InputPortWidth=2  Indices=[2]
  Sum7 : Sum  Inputs=|+-
  Sum9 : Sum
  Commanded Velocity [rad/s] [back front] : Outport
  wires:
  Kp_SEA_Trajectory/1 -> Product1/2
  Sum9/1 -> Commanded Velocity [rad/s] [back front]/1
  Measured Velocity [rad/s] [back front]/1 -> Selector7/1, Selector3/1
  Desired Velocity [rad/s] [back front]/1 -> Selector6/1, Selector2/1, Sum9/2
  Measured Position [rad] [back front]/1 -> Selector4/1, Selector/1, Sum7/2
  Sum7/1 -> Product1/1
  Product1/1 -> Sum9/1
  Mux12/1 -> Back Tracking/2
  Mux13/1 -> Back Tracking/1
  Desired Position [rad] [back front]/1 -> Selector5/1, Selector1/1, Sum7/1
  Mux1/1 -> Front Tracking/2
  Mux2/1 -> Front Tracking/1
  Selector/1 -> Mux13/1
  Selector1/1 -> Mux13/2
  Selector2/1 -> Mux12/1
  Selector3/1 -> Mux12/2
  Selector5/1 -> Mux2/2
  Selector4/1 -> Mux2/1
  Selector6/1 -> Mux1/1
  Selector7/1 -> Mux1/2

== system vertical_smm_3d_with_xz_lqr/Control/Behavior Control/Secondary Leg Behavior/Lowpass Filter (Swing) ==
  In : Inport
  Generated Filter Block : dsparch4/Biquad Filter  Tag=BlockMethodSubSystem  IIRFiltStruct=Direct form II  CoeffSource=Specify via dialog  BiQuadCoeffs=[1.0218648663828083 -2 1.0218648663828083 1 -1.9114378222117407 0.91557643487411833]  a0Flag=Warning  IC=0  ICnum=0  ICden=0  denAccumFracLength=30  denProdOutputFracLength=30  secondMemoryFracLength=15  roundingMode=Floor  overflowMode=off  ScaleValues=[0.0041174265739107223;22.985401576126357]  optimizeScaleValues=off  ScaleValueMode=Specify via input port (g)  scaleValueFracLength=14  FilterSource=Specify via dialog  FilterObject=Hm_biquad
  Out : Outport
  wires:
  In/1 -> Generated Filter Block/1
  Generated Filter Block/1 -> Out/1

== system vertical_smm_3d_with_xz_lqr/Control/Behavior Control/State Estimation/Kalman Filtering ==
  "COM from Left Foot [body, yawed, global]" : Inport  SampleTime=sample_time
  "COM from Right Foot [body, yawed, global]" : Inport  Port=2  SampleTime=sample_time
  GRFx [N] : Inport  Port=3  SampleTime=sample_time
  GRFy [N] : Inport  Port=4  SampleTime=sample_time
  GRFz [N] : Inport  Port=5  SampleTime=sample_time
  Right Vertical GRF [N] : Inport  Port=6  SampleTime=sample_time
  Left Vertical GRF [N] : Inport  Port=7  SampleTime=sample_time
  "Initial [x, dx, ddx] [m, m/s, m/s^2]" : Inport  Port=8  PortDimensions=3  SampleTime=sample_time
  "Initial [y, dy, ddy] [m, m/s, m/s^2]" : Inport  Port=9  PortDimensions=3  SampleTime=sample_time
  "Initial [z, dz, ddz] [m m/s m/s^2]" : Inport  Port=10  PortDimensions=3  SampleTime=sample_time
  COM XYZ Acceleration [m/s^2] x3 : Inport  Port=11  SampleTime=sample_time
  Entering Stance [1/0] : Inport  Port=12  PortDimensions=1  SampleTime=sample_time
  Enable : EnablePort  StatesWhenEnabling=reset
  Difference : simulink/Discrete/Difference  ICPrevInput=0.0  InputProcessing=Inherited  OutMin=[]  OutMax=[]  OutDataType=fixdt(1, 16)  OutScaling=2^-10  DoSatur=off
  Difference1 : simulink/Discrete/Difference  ICPrevInput=0.0  InputProcessing=Inherited  OutMin=[]  OutMax=[]  OutDataType=fixdt(1, 16)  OutScaling=2^-10  DoSatur=off
  Difference2 : simulink/Discrete/Difference  ICPrevInput=0.0  InputProcessing=Inherited  OutMin=[]  OutMax=[]  OutDataType=fixdt(1, 16)  OutScaling=2^-10  DoSatur=off
  Logical Operator : Logic  Operator=NOT  AllPortsSameDT=off  OutDataTypeStr=boolean
  Measurement Noise Covariance Matricies : MATLAB Function  TreatAsAtomicUnit=on
  Mux : Mux  Inputs=3
  Mux1 : Mux  Inputs=3
  Mux3 : Mux  Inputs=3
  P0_kalman_transverse : Constant  Value=P0_kalman_transverse
  P0_kalman_transverse1 : Constant  Value=P0_kalman_transverse
  P0_kalman_vertical : Constant  Value=P0_kalman_vertical
  Product : Product
  Product1 : Product
  Product2 : Product
  X State Kalman Filter : ctrlSharedLib/Kalman Filter  TimeDomain=Discrete-Time  UseCurrentEstimator=on  ModelSource=Individual A, B, C, D matrices  ModelSourceVariable=A_kf  A=A_kalman_transverse  B=B_kalman_transverse  C=C_kalman_transverse  D=0  NumberOfStates=2  NumberOfInputs=1  NumberOfOutputs=2  InitialEstimateSource=Input port  X0=initial_dx_estimate  P0=P0_kalman_transverse  UseK=off  UseGH=on  NumberOfProcessNoiseInputs=1  G=G_kalman_transverse  TimeInvariantG=on  H=0  TimeInvariantH=on  Q=Q_kalman_GRF_difference  TimeInvariantQ=on  R=1  TimeInvariantR=off  N=0  TimeInvariantN=on  AddInputPort=on  AddEnablePort=off  ExternalReset=Rising  OutputEstimatedY=off  OutputP=on  Ts=sample_time
  Y State Kalman Filter : ctrlSharedLib/Kalman Filter  TimeDomain=Discrete-Time  UseCurrentEstimator=on  ModelSource=Individual A, B, C, D matrices  ModelSourceVariable=A_kf  A=A_kalman_transverse  B=B_kalman_transverse  C=C_kalman_transverse  D=0  NumberOfStates=2  NumberOfInputs=1  NumberOfOutputs=2  InitialEstimateSource=Input port  X0=initial_dy_estimate  P0=P0_kalman_transverse  UseK=off  UseGH=on  NumberOfProcessNoiseInputs=1  G=G_kalman_transverse  TimeInvariantG=on  H=0  TimeInvariantH=on  Q=Q_kalman_GRF_difference  TimeInvariantQ=on  R=1  TimeInvariantR=off  N=0  TimeInvariantN=on  AddInputPort=on  AddEnablePort=off  ExternalReset=Rising  OutputEstimatedY=off  OutputP=on  Ts=sample_time
  Z State Kalman Filter : ctrlSharedLib/Kalman Filter  TimeDomain=Discrete-Time  UseCurrentEstimator=on  ModelSource=Individual A, B, C, D matrices  ModelSourceVariable=A_kf  A=A_kalman_vertical  B=B_kalman_vertical  C=C_kalman_vertical  D=0  NumberOfStates=2  NumberOfInputs=1  NumberOfOutputs=2  InitialEstimateSource=Input port  X0=[initial_z_estimate; initial_dz_estimate]  P0=P0_kalman_vertical  UseK=off  UseGH=on  NumberOfProcessNoiseInputs=1  G=G_kalman_vertical  TimeInvariantG=on  H=0  TimeInvariantH=on  Q=Q_kalman_GRF_difference  TimeInvariantQ=on  R=1  TimeInvariantR=off  N=0  TimeInvariantN=on  AddInputPort=on  AddEnablePort=off  OutputEstimatedY=off  OutputP=on  Ts=sample_time
  eigen values : MATLAB Function  TreatAsAtomicUnit=on
  eigen values1 : MATLAB Function  TreatAsAtomicUnit=on
  eigen values2 : MATLAB Function  TreatAsAtomicUnit=on
  left x yawed : Selector  InputPortWidth=9  Indices=[4]
  left y yawed : Selector  InputPortWidth=9  Indices=[5]
  left z yawed : Selector  InputPortWidth=9  Indices=[6]
  right x yawed : Selector  InputPortWidth=9  Indices=[4]
  right y yawed : Selector  InputPortWidth=9  Indices=[5]
  right z yawed : Selector  InputPortWidth=9  Indices=[6]
  x acceleration : Selector  InputPortWidth=3  Indices=[1]
  y acceleration : Selector  InputPortWidth=3  Indices=[2]
  z acceleration : Selector  InputPortWidth=3  Indices=[3]
  "[x, dx, ddx] [m/s, m/s^2]" : Outport
  "[y, dy, ddy] [m/s, m/s^2]" : Outport  Port=2
  "[z, dz, ddz] [m, m/s, m/s^2]" : Outport  Port=3
  "[x, dx, ddx] uncertainty" : Outport  Port=4
  "[y, dy, ddy] uncertainty" : Outport  Port=5
  "[z, dz, ddz] uncertainty" : Outport  Port=6
  wires:
  X State Kalman Filter/1 -> "[x, dx, ddx] [m/s, m/s^2]"/1
  eigen values1/1(E) -> "[y, dy, ddy] uncertainty"/1
  eigen values2/1(E) -> "[x, dx, ddx] uncertainty"/1
  Y State Kalman Filter/1 -> "[y, dy, ddy] [m/s, m/s^2]"/1
  y acceleration/1 -> Mux1/3
  x acceleration/1 -> Mux/3
  z acceleration/1 -> Mux3/3
  COM XYZ Acceleration [m/s^2] x3/1 -> z acceleration/1, y acceleration/1, x acceleration/1
  Z State Kalman Filter/1 -> "[z, dz, ddz] [m, m/s, m/s^2]"/1
  GRFy [N]/1 -> Difference1/1
  Mux3/1 -> Z State Kalman Filter/2  "yawed [left z, right z, ddz]"
  GRFx [N]/1 -> Difference2/1
  Measurement Noise Covariance Matricies/2(R_vertical) -> Z State Kalman Filter/5
  Measurement Noise Covariance Matricies/1(R_transverse) -> X State Kalman Filter/6, Y State Kalman Filter/6
  Mux1/1 -> Y State Kalman Filter/2  "yawed [left y, right y, ddy]"
  Mux/1 -> X State Kalman Filter/2  "yawed [left x, right x, ddx]"
  Right Vertical GRF [N]/1 -> Measurement Noise Covariance Matricies/2(vertical_GRF_R)
  Left Vertical GRF [N]/1 -> Measurement Noise Covariance Matricies/1(vertical_GRF_L)
  "COM from Left Foot [body, yawed, global]"/1 -> left z yawed/1, left y yawed/1, left x yawed/1
  left x yawed/1 -> Mux/1
  "COM from Right Foot [body, yawed, global]"/1 -> right z yawed/1, right y yawed/1, right x yawed/1
  right x yawed/1 -> Mux/2
  left y yawed/1 -> Mux1/1
  right y yawed/1 -> Mux1/2
  left z yawed/1 -> Mux3/1
  right z yawed/1 -> Mux3/2
  P0_kalman_transverse/1 -> X State Kalman Filter/4
  "Initial [x, dx, ddx] [m, m/s, m/s^2]"/1 -> X State Kalman Filter/3
  P0_kalman_transverse1/1 -> Y State Kalman Filter/4
  "Initial [y, dy, ddy] [m, m/s, m/s^2]"/1 -> Y State Kalman Filter/3
  P0_kalman_vertical/1 -> Z State Kalman Filter/4
  "Initial [z, dz, ddz] [m m/s m/s^2]"/1 -> Z State Kalman Filter/3
  X State Kalman Filter/2 -> eigen values2/1(Z)
  Y State Kalman Filter/2 -> eigen values1/1(Z)
  Z State Kalman Filter/2 -> eigen values/1(Z)
  eigen values/1(E) -> "[z, dz, ddz] uncertainty"/1
  Logical Operator/1 -> Product2/1, Product/1, Product1/1
  Difference/1 -> Product/2
  Entering Stance [1/0]/1 -> Y State Kalman Filter/5, X State Kalman Filter/5, Logical Operator/1
  Difference1/1 -> Product1/2
  Difference2/1 -> Product2/2
  Product2/1 -> X State Kalman Filter/1
  Product1/1 -> Y State Kalman Filter/1
  Product/1 -> Z State Kalman Filter/1
  GRFz [N]/1 -> Difference/1

== system vertical_smm_3d_with_xz_lqr/Control/Behavior Control/State Estimation/Lowpass Filter ==
  In : Inport
  Generated Filter Block : dsparch4/Biquad Filter  Tag=BlockMethodSubSystem  IIRFiltStruct=Direct form II  CoeffSource=Specify via dialog  BiQuadCoeffs=[1.0218648663828083 -2 1.0218648663828083 1 -1.9114378222117407 0.91557643487411833]  a0Flag=Warning  IC=0  ICnum=0  ICden=0  denAccumFracLength=30  denProdOutputFracLength=30  secondMemoryFracLength=15  roundingMode=Floor  overflowMode=off  ScaleValues=[0.0041174265739107223;22.985401576126357]  optimizeScaleValues=off  ScaleValueMode=Specify via input port (g)  scaleValueFracLength=14  FilterSource=Specify via dialog  FilterObject=Hm_biquad
  Out : Outport
  wires:
  In/1 -> Generated Filter Block/1
  Generated Filter Block/1 -> Out/1

== system vertical_smm_3d_with_xz_lqr/Control/Actuator Control with Torque SEA commands/Contact Velocities/Velocity on Contact/Subsystem ==
  in : Inport
  Enable : EnablePort
  out : Outport
  wires:
  in/1 -> out/1

== system vertical_smm_3d_with_xz_lqr/Control/Actuator Control with Torque SEA commands/Contact Velocities/Velocity on Contact1/Subsystem ==
  in : Inport
  Enable : EnablePort
  out : Outport
  wires:
  in/1 -> out/1

== system vertical_smm_3d_with_xz_lqr/Control/Actuator Control with Torque SEA commands/Contact Velocities/Velocity on Contact2/Subsystem ==
  in : Inport
  Enable : EnablePort
  out : Outport
  wires:
  in/1 -> out/1

== system vertical_smm_3d_with_xz_lqr/Control/Actuator Control with Torque SEA commands/Contact Velocities/Velocity on Contact3/Subsystem ==
  in : Inport
  Enable : EnablePort
  out : Outport
  wires:
  in/1 -> out/1

== system vertical_smm_3d_with_xz_lqr/Control/Actuator Control with Torque SEA commands/Timers/Time on Contact/Subsystem ==
  in : Inport
  Enable : EnablePort
  out : Outport
  wires:
  in/1 -> out/1

== system vertical_smm_3d_with_xz_lqr/Control/Actuator Control with Torque SEA commands/Timers/Time on Contact1/Subsystem ==
  in : Inport
  Enable : EnablePort
  out : Outport
  wires:
  in/1 -> out/1

== system vertical_smm_3d_with_xz_lqr/Control/Actuator Control with Torque SEA commands/Timers/Time on Contact2/Subsystem ==
  in : Inport
  Enable : EnablePort
  out : Outport
  wires:
  in/1 -> out/1

== system vertical_smm_3d_with_xz_lqr/Control/Actuator Control with Torque SEA commands/Timers/Time on Contact3/Subsystem ==
  in : Inport
  Enable : EnablePort
  out : Outport
  wires:
  in/1 -> out/1

== system vertical_smm_3d_with_xz_lqr/Control/Behavior Control/Primary and Lateral Behavior/Circular Buffer/Enabled on Touchdown ==
  In : Inport
  Enable : EnablePort
  Out : Outport
  wires:
  In/1 -> Out/1

== system vertical_smm_3d_with_xz_lqr/Control/Behavior Control/Primary and Lateral Behavior/Flight/Back//Front PD ==
  Desired Position [rad] [back front] : Inport
  Desired Velocity [rad/s] [back front] : Inport  Port=2
  Measured Position [rad] [back front] : Inport  Port=3
  Measured Velocity [rad/s] [back front] : Inport  Port=4
  Back Tracking : Scope  NumInputPorts=2
      settings: YMin=3.725~-1  YMax=4.05~0.9  SaveName=ScopeData6  SampleInput=on
  Front Tracking : Scope  NumInputPorts=2
      settings: YMin=-1~-0.8  YMax=1~1.4  SaveName=ScopeData31  SampleInput=on
  Kp_SEA_Trajectory : Constant  Value=kp_velocity_swing_trajectory
  Mux{1..2,12..13} (4 alike) : Mux  Inputs=2
  Product1 : Product
  Selector{,1..3} (4 alike) : Selector  InputPortWidth=2  Indices=[1]
  Selector{4..7} (4 alike) : Selector  InputPortWidth=2  Indices=[2]
  Sum7 : Sum  Inputs=|+-
  Sum9 : Sum
  Commanded Velocity [rad/s] [back front] : Outport
  wires:
  Kp_SEA_Trajectory/1 -> Product1/2
  Sum9/1 -> Commanded Velocity [rad/s] [back front]/1
  Measured Velocity [rad/s] [back front]/1 -> Selector7/1, Selector3/1
  Desired Velocity [rad/s] [back front]/1 -> Selector6/1, Selector2/1, Sum9/2
  Measured Position [rad] [back front]/1 -> Selector4/1, Selector/1, Sum7/2
  Sum7/1 -> Product1/1
  Product1/1 -> Sum9/1
  Mux12/1 -> Back Tracking/2
  Mux13/1 -> Back Tracking/1
  Desired Position [rad] [back front]/1 -> Selector5/1, Selector1/1, Sum7/1
  Mux1/1 -> Front Tracking/2
  Mux2/1 -> Front Tracking/1
  Selector/1 -> Mux13/1
  Selector1/1 -> Mux13/2
  Selector2/1 -> Mux12/1
  Selector3/1 -> Mux12/2
  Selector5/1 -> Mux2/2
  Selector4/1 -> Mux2/1
  Selector6/1 -> Mux1/1
  Selector7/1 -> Mux1/2

== system vertical_smm_3d_with_xz_lqr/Control/Behavior Control/Primary and Lateral Behavior/Flight/Hold Values on Takeoff ==
  in : Inport
  Trigger : TriggerPort  ShowOutputPort=on  PortDimensions=1
  Subsystem : Subsystem
  out : Outport
  wires:
  in/1 -> Subsystem/1(in)
  Subsystem/1(out) -> out/1
  Trigger/1 -> Subsystem/Enable

== system vertical_smm_3d_with_xz_lqr/Control/Behavior Control/Primary and Lateral Behavior/Stance/Chirp Frequency ==
  Time Since Stance : Inport
  Chirp Freq Factor Saturation : Saturate  UpperLimit=standing_bounce_max_chirp_scale  LowerLimit=0
      settings: AttributesFormatString=Top: %<UpperLimit>\nBottom: %<LowerLimit>
  Compare To Constant1 : simulink/Logic and Bit Operations/Compare To Constant  relop=~=  const=standing_bounce_max_chirp_scale  OutDataTypeStr=boolean
  Constant1 : Constant
  Constant5 : Constant  Value=standing_bounce_increase_rate
  Product{1..4} (4 alike) : Product
  Sum : Sum  Inputs=++|
  standing_bounce_frequency : Constant  Value=standing_bounce_frequency
  w : Outport
  dw/dt : Outport  Port=2
  wires:
  standing_bounce_frequency/1 -> Product2/1, Product3/1
  Chirp Freq Factor Saturation/1 -> Product3/2, Compare To Constant1/1
  Product3/1 -> w/1
  Product1/1 -> dw/dt/1
  Compare To Constant1/1 -> Product1/1
  Product2/1 -> Product1/2
  Constant5/1 -> Product2/2, Product4/2
  Time Since Stance/1 -> Product4/1
  Sum/1 -> Chirp Freq Factor Saturation/1
  Product4/1 -> Sum/2
  Constant1/1 -> Sum/1

== system vertical_smm_3d_with_xz_lqr/Control/Behavior Control/Primary and Lateral Behavior/Stance/Compute Forces1 ==
  XYZ Acceleration : Inport
  Constant5 : Constant  Value=g
  Demux : Demux  Outputs=3
  Gain4 : Gain  Gain=m_total_real
  Mux : Mux  Inputs=3
  Sum8 : Sum  Inputs=|++
  XYZ Force : Outport
  wires:
  Constant5/1 -> Sum8/2
  XYZ Acceleration/1 -> Demux/1
  Gain4/1 -> XYZ Force/1
  Mux/1 -> Gain4/1
  Sum8/1 -> Mux/3
  Demux/3 -> Sum8/1
  Demux/2 -> Mux/2
  Demux/1 -> Mux/1

== system vertical_smm_3d_with_xz_lqr/Control/Behavior Control/Primary and Lateral Behavior/Stance/Hold Values on Takeoff ==
  in : Inport
  Trigger : TriggerPort  ShowOutputPort=on  PortDimensions=1
  Subsystem : Subsystem
  out : Outport
  wires:
  Trigger/1 -> Subsystem/Enable
  Subsystem/1(out) -> out/1
  in/1 -> Subsystem/1(in)

== system vertical_smm_3d_with_xz_lqr/Control/Behavior Control/Primary and Lateral Behavior/Stance/Hold Values on Touchdown ==
  in : Inport
  Trigger : TriggerPort  ShowOutputPort=on  PortDimensions=1
  Subsystem : Subsystem
  out : Outport
  wires:
  in/1 -> Subsystem/1(in)
  Subsystem/1(out) -> out/1
  Trigger/1 -> Subsystem/Enable
